simulink model "xindiandao030406"  (R2019a)
settings: Solver=VariableStepAuto  StartTime=0.0  StopTime=10  RelTol=1e-3
libraries: commanapbnd3 x1
settings Model: Creator=Zezzid  LastModifiedBy=Zezzid

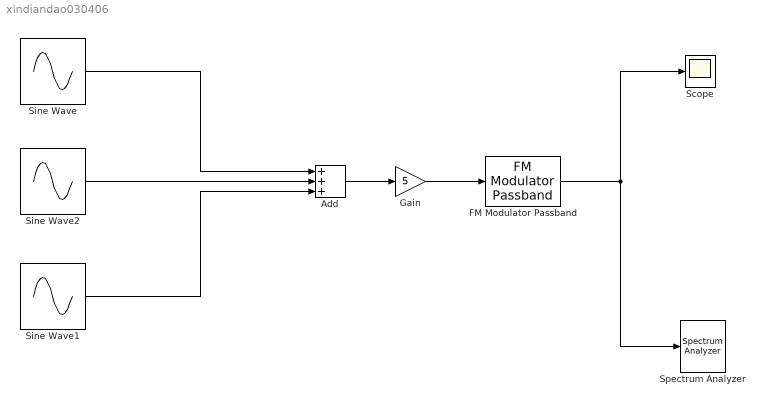
== system xindiandao030406 ==
  Add : Sum  Inputs=+++
  FM Modulator Passband : commanapbnd3/FM Modulator Passband  Fc=300  Ph=0  Kc=50
      settings: SourceProductName=Communications Toolbox  SourceProductBaseCode=CM
  Gain : Gain  Gain=5
  Scope : Scope
  Sine Wave : Sin  Amplitude=0.3  Frequency=2*pi*10  SampleTime=1/3000
  Sine Wave1 : Sin  Amplitude=0.5  Frequency=2*pi*30  Phase=pi/3  SampleTime=1/3000
  Sine Wave2 : Sin  Amplitude=0.2  Frequency=2*pi*20  Phase=pi/6  SampleTime=1/3000
  Spectrum Analyzer : SpectrumAnalyzer
  wires:
  Sine Wave/1 -> Add/1
  Sine Wave2/1 -> Add/2
  Sine Wave1/1 -> Add/3
  Add/1 -> Gain/1
  Gain/1 -> FM Modulator Passband/1
  FM Modulator Passband/1 -> Spectrum Analyzer/1, Scope/1
